simulink model "problem_6_5"  (R2018a)
settings: Solver=FixedStepDiscrete  StartTime=0.0  StopTime=0.05  FixedStep=1e-5  RelTol=1e-3
undefined symbols (not defined in the file or in its folder): get
libraries: dspobslib x4, dspxfrm3 x2, dspsigops x2
settings Model: Creator=Ryan  LastModifiedBy=Ryan

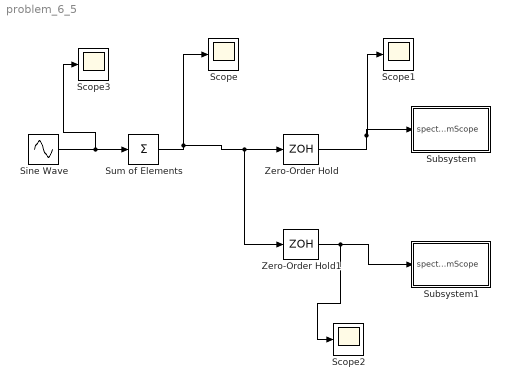
== system problem_6_5 ==
  Scope{,1..3} (4 alike) : Scope
  Sine Wave : Sin  Frequency=2*pi*[0.9,1.1]*1e3  Samples=2*pi*[.9,1.1]*1e3;  SampleTime=0
  Subsystem : Subsystem
  Subsystem1 : Subsystem
  Sum of Elements : Sum  Inputs=+
  Zero-Order Hold : ZeroOrderHold  SampleTime=5e-5
  Zero-Order Hold1 : ZeroOrderHold  SampleTime=20e-5
  wires:
  Zero-Order Hold/1 -> Scope1/1, Subsystem/1(spectrumScope)
  Zero-Order Hold1/1 -> Scope2/1, Subsystem1/1(spectrumScope)
  Sine Wave/1 -> Scope3/1, Sum of Elements/1
  Sum of Elements/1 -> Zero-Order Hold1/1, Zero-Order Hold/1, Scope/1

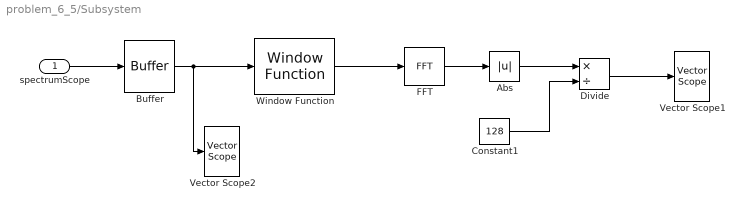
== system problem_6_5/Subsystem ==
  spectrumScope : Inport
  Abs : Abs
  Buffer : Buffer  N=128  OutputFrames=off
  Constant1 : Constant  Value=128
  Divide : Product  Inputs=*/
  FFT : dspxfrm3/FFT  FFTImplementation=Auto  CompMethod=Table lookup  TableOpt=NEW  TableOptActive=Speed  BitRevOrder=off  Normalize=off  InheritFFTLength=on  FFTLength=64  WrapInput=on  roundingMode=Floor  overflowMode=off  firstCoeffDataTypeStr=Inherit: Same word length as input  firstCoeffLastDataTypeStr=Inherit: Same word length as input  outputMin=[]  outputMax=[]
  Vector Scope1 : dspobslib/Vector Scope  ScopeProperties=on  Domain=Frequency  HorizSpan=1  DisplayProperties=off  AxisGrid=on  Memory=off  FrameNumber=on  AxisLegend=off  AxisZoom=off  OpenScopeAtSimStart=on  OpenScopeImmediately=off  FigPos=get(0,'defaultfigureposition')  AxisProperties=off  XUnits=Hertz  XRange=[0...Fs/2]  InheritXIncr=on  XIncr=1  XLabel=Time  XLimit=Auto  XMin=0  XMax=1  XStart=0  YUnits=dB  YLabel=Amplitude  LineProperties=off  LineMarkers=.  XAxisParamsVer=6.9
      settings: SourceProductName=DSP System Toolbox  SourceProductBaseCode=DS  YMin=-160  YMax=1
  Vector Scope2 : dspobslib/Vector Scope  ScopeProperties=on  Domain=Time  HorizSpan=1  DisplayProperties=off  AxisGrid=on  Memory=off  FrameNumber=on  AxisLegend=off  AxisZoom=off  OpenScopeAtSimStart=on  OpenScopeImmediately=off  FigPos=get(0,'defaultfigureposition')  AxisProperties=off  XUnits=Hertz  XRange=[0...Fs/2]  InheritXIncr=on  XIncr=1  XLabel=Time  XLimit=Auto  XMin=0  XMax=1  XStart=0  YUnits=dB  YLabel=Amplitude  LineProperties=off  LineMarkers=.  XAxisParamsVer=6.9
      settings: SourceProductName=DSP System Toolbox  SourceProductBaseCode=DS  YMin=-3  YMax=3
  Window Function : dspsigops/Window Function  winmode=Apply window to input  wintype=Hann  sampmode=Continuous  samptime=1  N=64  Rs=50  beta=10  winsamp=Symmetric  UserWindow=hamming  OptParams=off  UserParams={'symmetric'}  dataType=double  isSigned=on  wordLen=16  udDataType=sfix(16)  fracBitsMode=Best precision  numFracBits=15  roundingMode=Floor  overflowMode=off  numSidelobes=4  sidelobeLevel=-30
      settings: SourceProductName=DSP System Toolbox  SourceProductBaseCode=DS
  wires:
  Abs/1 -> Divide/1
  Constant1/1 -> Divide/2
  Divide/1 -> Vector Scope1/1
  Buffer/1 -> Vector Scope2/1, Window Function/1
  FFT/1 -> Abs/1
  spectrumScope/1 -> Buffer/1
  Window Function/1 -> FFT/1

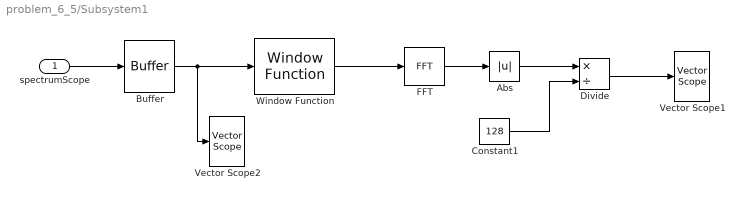
== system problem_6_5/Subsystem1 ==
  spectrumScope : Inport
  Abs : Abs
  Buffer : Buffer  N=128  OutputFrames=off
  Constant1 : Constant  Value=128
  Divide : Product  Inputs=*/
  FFT : dspxfrm3/FFT  FFTImplementation=Auto  CompMethod=Table lookup  TableOpt=NEW  TableOptActive=Speed  BitRevOrder=off  Normalize=off  InheritFFTLength=on  FFTLength=64  WrapInput=on  roundingMode=Floor  overflowMode=off  firstCoeffDataTypeStr=Inherit: Same word length as input  firstCoeffLastDataTypeStr=Inherit: Same word length as input  outputMin=[]  outputMax=[]
  Vector Scope1 : dspobslib/Vector Scope  ScopeProperties=on  Domain=Frequency  HorizSpan=1  DisplayProperties=off  AxisGrid=on  Memory=off  FrameNumber=on  AxisLegend=off  AxisZoom=off  OpenScopeAtSimStart=on  OpenScopeImmediately=off  FigPos=get(0,'defaultfigureposition')  AxisProperties=off  XUnits=Hertz  XRange=[0...Fs/2]  InheritXIncr=on  XIncr=1  XLabel=Time  XLimit=Auto  XMin=0  XMax=1  XStart=0  YUnits=dB  YLabel=Amplitude  LineProperties=off  LineMarkers=.  XAxisParamsVer=6.9
      settings: SourceProductName=DSP System Toolbox  SourceProductBaseCode=DS  YMin=-160  YMax=1
  Vector Scope2 : dspobslib/Vector Scope  ScopeProperties=on  Domain=Time  HorizSpan=1  DisplayProperties=off  AxisGrid=on  Memory=off  FrameNumber=on  AxisLegend=off  AxisZoom=off  OpenScopeAtSimStart=on  OpenScopeImmediately=off  FigPos=get(0,'defaultfigureposition')  AxisProperties=off  XUnits=Hertz  XRange=[0...Fs/2]  InheritXIncr=on  XIncr=1  XLabel=Time  XLimit=Auto  XMin=0  XMax=1  XStart=0  YUnits=dB  YLabel=Amplitude  LineProperties=off  LineMarkers=.  XAxisParamsVer=6.9
      settings: SourceProductName=DSP System Toolbox  SourceProductBaseCode=DS  YMin=-3  YMax=3
  Window Function : dspsigops/Window Function  winmode=Apply window to input  wintype=Hann  sampmode=Continuous  samptime=1  N=64  Rs=50  beta=10  winsamp=Symmetric  UserWindow=hamming  OptParams=off  UserParams={'symmetric'}  dataType=double  isSigned=on  wordLen=16  udDataType=sfix(16)  fracBitsMode=Best precision  numFracBits=15  roundingMode=Floor  overflowMode=off  numSidelobes=4  sidelobeLevel=-30
      settings: SourceProductName=DSP System Toolbox  SourceProductBaseCode=DS
  wires:
  Window Function/1 -> FFT/1
  spectrumScope/1 -> Buffer/1
  FFT/1 -> Abs/1
  Buffer/1 -> Vector Scope2/1, Window Function/1
  Divide/1 -> Vector Scope1/1
  Constant1/1 -> Divide/2
  Abs/1 -> Divide/1
